simulink model "EarthmoverMechPT"  (Simulink 6.6)
settings: Solver=FixedStepDiscrete  StartTime=0  StopTime=100  FixedStep=0.01  MaxStep=0.01  RelTol=1e-12
undefined symbols (not defined in the file or in its folder): engineM, slippageM
libraries: simulink x17
settings Model: Creator=Messer  LastModifiedBy=Messer
settings SolverCC: SolverResetMethod=Robust
settings DebuggingCC: AlgebraicLoopMsg=none  SignalResolutionControl=TryResolveAllWithWarning  MultiTaskDSMMsg=warning  MultiTaskCondExecSysMsg=none  StrictBusMsg=None
settings RTWCC: IncludeERTFirstTime=on

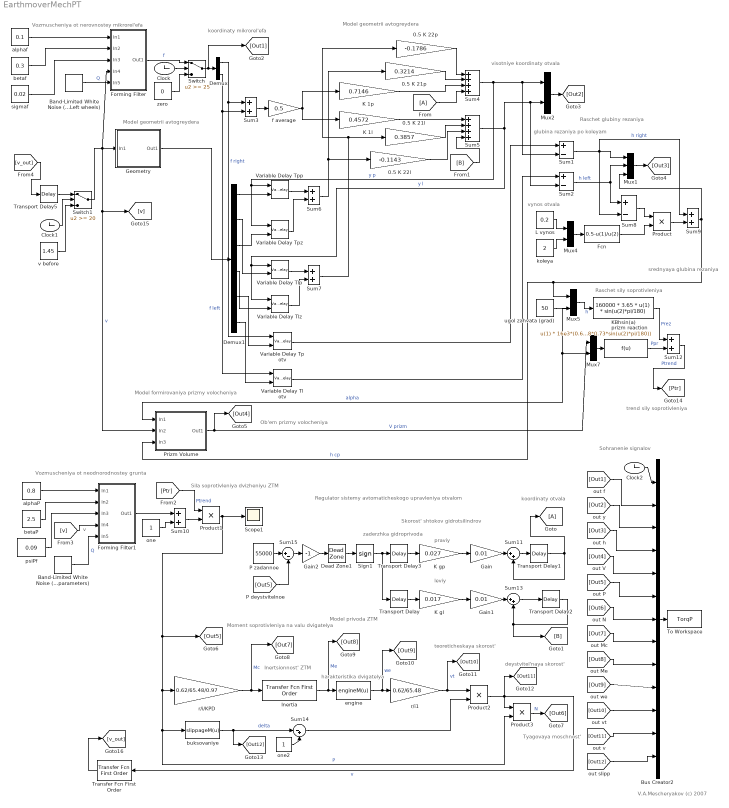
== system EarthmoverMechPT ==
  note: v
  note: V.A.Mescheryakov (c) 2007
  note: Sohranenie signalov
  note: Regulator sistemy
      | avtomaticheskogo upravleniya otvalom
  note: Skorost' shtokov
      | gidrotsilindrov
  note: praviy
  note: leviy
  note: zaderzhka
      | gidroprivoda
  note: Sila soprotivleniya
      | dvizheniyu ZTM
  note: harakteristika
      | dvigatelya
  note: Inertsionnost' ZTM
  note: Moment soprotivleniya
      | na valu dvigatelya
  note: Vozmuscheniya ot neodnorodnostey grunta
  note: teoreticheskaya skorost'
  note: deystvitel'naya skorost'
  note: koordinaty otvala
  note: Vozmuscheniya ot nerovnostey mikrorel'efa
  note: visotniye koordinaty otvala
  note: glubina rezaniya
      | po koleyam
  note: srednyaya
      | glubina
      | rezaniya
  note: vynos otvala
  note: trend sily soprotivleniya
  note: Ob'em prizmy volocheniya
  note: Model formirovaniya prizmy volocheniya
  note: Model geometrii avtogreydera
  note: Model geometrii avtogreydera
  note: koordinaty mikrorel'efa
  note: Model privoda ZTM
  note: Tyagovaya
      | moschnost'
  note: Raschet glubiny rezaniya
  note: Raschet sily soprotivleniya
  0.5 K 21l : Gain  Gain=0.3857
  0.5 K 21p : Gain  Gain=0.3214
  0.5 K 22l : Gain  Gain=-0.1143
  0.5 K 22p : Gain  Gain=-0.1786
  Band-Limited White Noise (Right & Left wheels) : simulink/Sources/Band-Limited White Noise  SystemSampleTime=-1  Cov=[1 1]  Ts=0.01  seed=[1111 2111]  VectorParams1D=off
  Band-Limited White Noise (Soil parameters) : simulink/Sources/Band-Limited White Noise  SystemSampleTime=-1  Cov=[1]  Ts=0.01  seed=[1112]
  Bus Creator2 : BusCreator  Inputs=13
  Clock : Clock
      settings: Decimation=10
  Clock1 : Clock
      settings: Decimation=10
  Clock2 : Clock
      settings: Decimation=10
  Dead Zone1 : DeadZone  LowerValue=-700  UpperValue=700  SaturateOnIntegerOverflow=on
  Demux : Demux  Outputs=2
  Demux1 : Demux  Outputs=6
  Fcn : Fcn  Expr=0.5-u(1)/u(2)
  Forming Filter : Subsystem
  Forming Filter1 : Subsystem
  Gain : Gain  Gain=0.01
  Gain1 : Gain  Gain=0.01
  Gain2 : Gain  Gain=-1
  Geometry : Subsystem
  Inertia : simulink/Discrete/Transfer Fcn First Order  SystemSampleTime=-1  PoleZ=exp(-1/0.48*0.01)  ICPrevOutput=0  DoSatur=off
  K 1l : Gain  Gain=0.4572
  K 1p : Gain  Gain=0.7146
  K gl : Gain  Gain=0.017
  K gp : Gain  Gain=0.027
  KBhsin(a) : Fcn  Expr=160000 * 3.65 * u(1) * sin(u(2)*pi/180)
  L vynos : Constant  Value=0.2
  Mux1 : Mux  Inputs=3
  Mux{2,4..5,7} (4 alike) : Mux  Inputs=2
  P zadannoe : Constant  Value=55000
  Prizm Volume : Subsystem
  Product{,1..3} (4 alike) : Product  RndMeth=Zero
  Scope1 : Scope
      settings: YMin=0  YMax=75000  SaveName=cr1  DataFormat=Array
  Sign1 : Signum
  Sum1 : Sum  Inputs=+-
  Sum{3,6..7,9..10,12} (6 alike) : Sum
  Sum11 : Sum  Inputs=|++
  Sum13 : Sum  Inputs=|++
  Sum14 : Sum  Inputs=|-+
  Sum15 : Sum  Inputs=|+-
  Sum2 : Sum  Inputs=+-
  Sum4 : Sum  Inputs=++++
  Sum5 : Sum  Inputs=++++
  Sum8 : Sum  Inputs=+-
  Switch : Switch  Threshold=25  ZeroCross=off
  Switch1 : Switch  Threshold=20  ZeroCross=off
  To Workspace : ToWorkspace  VariableName=TorqP  SampleTime=-1  SaveFormat=Array
  Transfer Fcn First Order : simulink/Discrete/Transfer Fcn First Order  Orientation=left  SystemSampleTime=-1  PoleZ=0.99  ICPrevOutput=0  DoSatur=off
  Transport Delay : TransportDelay  DelayTime=0.1  InitialOutput=-1
  Transport Delay1 : TransportDelay  DelayTime=0.01
  Transport Delay2 : TransportDelay  DelayTime=0.01
  Transport Delay3 : TransportDelay  DelayTime=0.1  InitialOutput=-1
  Transport Delay5 : TransportDelay  DelayTime=0.01  InitialOutput=1
  Variable Delay Tl otv : VariableTransportDelay  MaximumDelay=20
  Variable Delay Tlp : VariableTransportDelay  MaximumDelay=20
  Variable Delay Tlz : VariableTransportDelay  MaximumDelay=20
  Variable Delay Tp otv : VariableTransportDelay  MaximumDelay=20
  Variable Delay Tpp : VariableTransportDelay  MaximumDelay=20
  Variable Delay Tpz : VariableTransportDelay  MaximumDelay=20
  alphaP : Constant  Value=0.8
  alphaf : Constant  Value=0.1
  betaP : Constant  Value=2.5
  betaf : Constant  Value=0.3
  buksovaniye : MATLABFcn  MATLABFcn=slippageM(u)  OutputDimensions=1
  engine : MATLABFcn  MATLABFcn=engineM(u)  OutputDimensions=1
  f average : Gain  Gain=0.5
  koleya : Constant  Value=2
  one : Constant
  one2 : Constant
  prizm reaction : Fcn  Expr=u(1) * 16e3*(0.65*sin(u(2)*pi/180)+0.65*0.73*cos(u(2)*pi/180)+0.5868*0.73*sin(u(2)*pi/180))
  psiPf : Constant  Value=0.09
  r/i/KPD : Gain  Gain=0.62/65.48/0.97
  r/i1 : Gain  Gain=0.62/65.48
  sigmaf : Constant  Value=0.02
  ugol zahvata (grad) : Constant  Value=50
  v before : Constant  Value=1.45
  zero : Constant  Value=0
  wires:
  Forming Filter/1(Out1) -> Switch/1  "f"
  alphaf/1 -> Forming Filter/1(In1)
  betaf/1 -> Forming Filter/2(In2)
  sigmaf/1 -> Forming Filter/3(In3)
  Switch1/1 -> Forming Filter/4(In4), Geometry/1(In1), [v], Prizm Volume/2(In2)  "v"
  f average/1 -> K 1p/1, K 1l/1
  Geometry/1(Out1) -> Demux1/1
  Demux1/1 -> Variable Delay Tpp/2
  Demux1/2 -> Variable Delay Tlp/2
  Demux1/3 -> Variable Delay Tpz/2
  Demux1/4 -> Variable Delay Tlz/2
  Demux1/5 -> Variable Delay Tp otv/2
  Demux1/6 -> Variable Delay Tl otv/2
  Sum4/1 -> Variable Delay Tpz/1, Variable Delay Tpp/1, Sum1/2, Mux2/1  "y p"
  Sum5/1 -> Variable Delay Tlz/1, Variable Delay Tlp/1, Mux2/2, Sum2/2  "y l"
  K 1l/1 -> Sum5/1
  K 1p/1 -> Sum4/3
  Variable Delay Tpp/1 -> Sum6/1
  Variable Delay Tpz/1 -> Sum6/2
  Variable Delay Tlp/1 -> Sum7/1
  Variable Delay Tlz/1 -> Sum7/2
  0.5 K 21p/1 -> Sum4/2
  0.5 K 21l/1 -> Sum5/2
  Sum6/1 -> 0.5 K 21p/1, 0.5 K 22l/1
  Sum7/1 -> 0.5 K 21l/1, 0.5 K 22p/1
  0.5 K 22p/1 -> Sum4/1
  0.5 K 22l/1 -> Sum5/3
  Variable Delay Tp otv/1 -> Sum1/1
  Variable Delay Tl otv/1 -> Sum2/1
  Mux2/1 -> [Out2]
  [A] -> Sum4/4
  Sum1/1 -> Mux1/1, Sum8/2, Sum9/1  "h right"
  Sum2/1 -> Mux1/2, Sum8/1  "h left"
  Mux1/1 -> [Out3]
  Sum3/1 -> f average/1
  Clock/1 -> Switch/2
  zero/1 -> Switch/3
  [B] -> Sum5/4
  L vynos/1 -> Mux4/1
  koleya/1 -> Mux4/2
  Mux4/1 -> Fcn/1
  Sum8/1 -> Product/1
  Fcn/1 -> Product/2
  Product/1 -> Sum9/2
  Sum9/1 -> Mux1/3, Mux5/1, Prizm Volume/3(In3)  "h cp"
  ugol zahvata (grad)/1 -> Mux5/2, Mux7/2, Prizm Volume/1(In1)  "alpha"
  Mux5/1 -> KBhsin(a)/1  "h"
  KBhsin(a)/1 -> Sum12/1  "Prez"
  prizm reaction/1 -> Sum12/2  "Ppr"
  Mux7/1 -> prizm reaction/1
  Band-Limited White Noise (Right & Left wheels)/1 -> Forming Filter/5(In5)  "Q"
  Switch/1 -> Demux/1, [Out1]
  Demux/1 -> Sum3/1, Variable Delay Tp otv/1  "f right"
  Demux/2 -> Sum3/2, Variable Delay Tl otv/1  "f left"
  Prizm Volume/1(Out1) -> Mux7/1, [Out4]  "V prizm"
  alphaP/1 -> Forming Filter1/1(In1)
  betaP/1 -> Forming Filter1/2(In2)
  psiPf/1 -> Forming Filter1/3(In3)
  Band-Limited White Noise (Soil parameters)/1 -> Forming Filter1/5(In5)  "Q"
  one/1 -> Sum10/2
  Forming Filter1/1(Out1) -> Sum10/1
  Sum10/1 -> Product1/2
  Product1/1 -> r/i/KPD/1, Product3/2, buksovaniye/1, [Out5], Scope1/1  "P"
  K gp/1 -> Gain/1
  K gl/1 -> Gain1/1
  r/i1/1 -> Product2/1, [Out10]  "vt"
  Product2/1 -> [Out11], Product3/1, Transfer Fcn First Order/1  "v"
  Product3/1 -> [Out6]  "N"
  one2/1 -> Sum14/2
  Sum14/1 -> Product2/2
  r/i/KPD/1 -> Inertia/1, [Out7]  "Mc"
  Clock1/1 -> Switch1/2
  v before/1 -> Switch1/3
  Bus Creator2/1 -> To Workspace/1
  Clock2/1 -> Bus Creator2/1
  [Out1] -> Bus Creator2/2
  [Out2] -> Bus Creator2/3
  [Out3] -> Bus Creator2/4
  [Out4] -> Bus Creator2/5
  [Out5] -> Bus Creator2/6
  [Out6] -> Bus Creator2/7
  [Out7] -> Bus Creator2/8
  [Out8] -> Bus Creator2/9
  [Out9] -> Bus Creator2/10
  [Out10] -> Bus Creator2/11
  [Out11] -> Bus Creator2/12
  [Out12] -> Bus Creator2/13
  Inertia/1 -> engine/1, [Out8]  "Me"
  buksovaniye/1 -> Sum14/1, [Out12]  "delta"
  engine/1 -> r/i1/1, [Out9]  "we"
  Gain/1 -> Sum11/1
  Sum11/1 -> Transport Delay1/1
  Transport Delay1/1 -> Sum11/2, [A]
  Gain1/1 -> Sum13/1
  Sum13/1 -> Transport Delay2/1
  Transport Delay2/1 -> Sum13/2, [B]
  Sum12/1 -> [Ptr]  "Ptrend"
  [Ptr] -> Product1/1  "Ptrend"
  [v] -> Forming Filter1/4(In4)
  [v_out] -> Transport Delay5/1
  Transfer Fcn First Order/1 -> [v_out]
  Transport Delay5/1 -> Switch1/1
  P zadannoe/1 -> Sum15/1
  Dead Zone1/1 -> Sign1/1
  Sign1/1 -> Transport Delay3/1, Transport Delay/1
  Transport Delay3/1 -> K gp/1
  Transport Delay/1 -> K gl/1
  [Out5] -> Sum15/2
  Gain2/1 -> Dead Zone1/1
  Sum15/1 -> Gain2/1

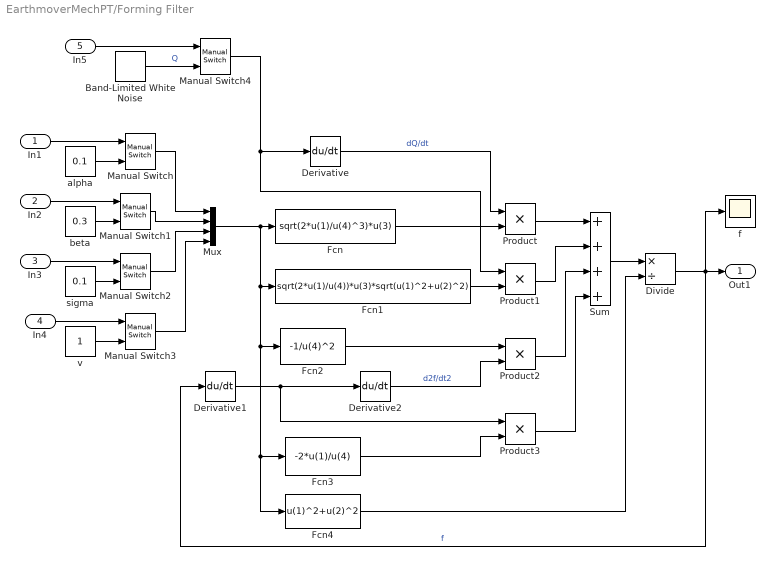
== system EarthmoverMechPT/Forming Filter ==
  In1 : Inport
  In2 : Inport  Port=2
  In3 : Inport  Port=3
  In4 : Inport  Port=4
  In5 : Inport  Port=5
  Band-Limited White Noise : simulink/Sources/Band-Limited White Noise  SystemSampleTime=-1  Cov=1  Ts=0.01  seed=[23341]
  Derivative : Derivative
  Derivative1 : Derivative
  Derivative2 : Derivative
  Divide : Product  Inputs=*/  OutScaling=2^-10
  Fcn : Fcn  Expr=sqrt(2*u(1)/u(4)^3)*u(3)
  Fcn1 : Fcn  Expr=sqrt(2*u(1)/u(4))*u(3)*sqrt(u(1)^2+u(2)^2)
  Fcn2 : Fcn  Expr=-1/u(4)^2
  Fcn3 : Fcn  Expr=-2*u(1)/u(4)
  Fcn4 : Fcn  Expr=u(1)^2+u(2)^2
  Manual Switch{,1..4} (5 alike) : simulink/Signal Routing/Manual Switch  SystemSampleTime=-1  sw=1  action=0  varsize=off
  Mux : Mux
  Product{,1..3} (4 alike) : Product  RndMeth=Zero
  Sum : Sum  Inputs=++++
  alpha : Constant  Value=0.1
  beta : Constant  Value=0.3
  f : Scope
      settings: SaveName=ScopeData12
  sigma : Constant  Value=0.1
  v : Constant
  Out1 : Outport
  wires:
  Mux/1 -> Fcn/1, Fcn1/1, Fcn3/1, Fcn4/1, Fcn2/1
  Derivative/1 -> Product/1  "dQ/dt"
  Fcn/1 -> Product/2
  Fcn1/1 -> Product1/2
  Product/1 -> Sum/1
  Product1/1 -> Sum/2
  Derivative1/1 -> Derivative2/1, Product3/1
  Derivative2/1 -> Product2/2  "d2f/dt2"
  Fcn2/1 -> Product2/1
  Product2/1 -> Sum/3
  Product3/1 -> Sum/4
  Fcn3/1 -> Product3/2
  Sum/1 -> Divide/1
  Fcn4/1 -> Divide/2
  Divide/1 -> Derivative1/1, f/1, Out1/1  "f"
  In1/1 -> Manual Switch/1
  alpha/1 -> Manual Switch/2
  Manual Switch/1 -> Mux/1
  In2/1 -> Manual Switch1/1
  beta/1 -> Manual Switch1/2
  Manual Switch1/1 -> Mux/2
  sigma/1 -> Manual Switch2/2
  In3/1 -> Manual Switch2/1
  Manual Switch2/1 -> Mux/3
  Manual Switch3/1 -> Mux/4
  In4/1 -> Manual Switch3/1
  v/1 -> Manual Switch3/2
  Band-Limited White Noise/1 -> Manual Switch4/2  "Q"
  In5/1 -> Manual Switch4/1
  Manual Switch4/1 -> Derivative/1, Product1/1

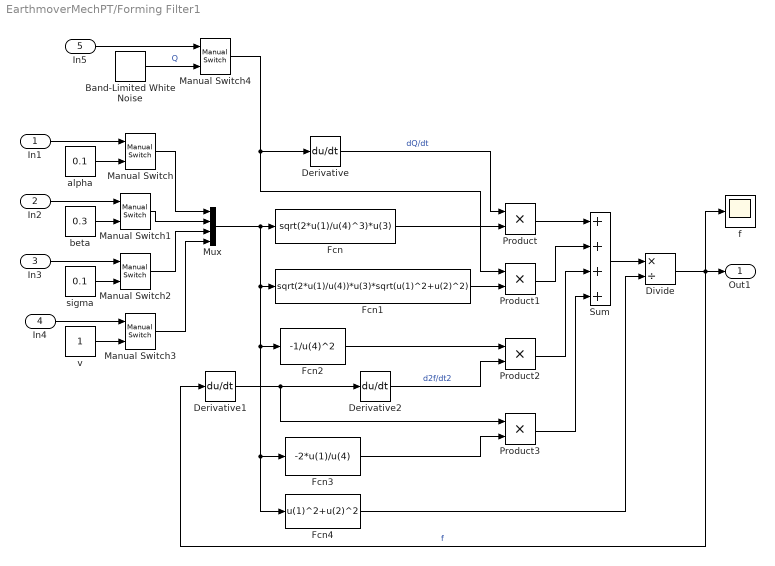
== system EarthmoverMechPT/Forming Filter1 ==
  In1 : Inport
  In2 : Inport  Port=2
  In3 : Inport  Port=3
  In4 : Inport  Port=4
  In5 : Inport  Port=5
  Band-Limited White Noise : simulink/Sources/Band-Limited White Noise  SystemSampleTime=-1  Cov=1  Ts=0.01  seed=[23341]
  Derivative : Derivative
  Derivative1 : Derivative
  Derivative2 : Derivative
  Divide : Product  Inputs=*/  OutScaling=2^-10
  Fcn : Fcn  Expr=sqrt(2*u(1)/u(4)^3)*u(3)
  Fcn1 : Fcn  Expr=sqrt(2*u(1)/u(4))*u(3)*sqrt(u(1)^2+u(2)^2)
  Fcn2 : Fcn  Expr=-1/u(4)^2
  Fcn3 : Fcn  Expr=-2*u(1)/u(4)
  Fcn4 : Fcn  Expr=u(1)^2+u(2)^2
  Manual Switch{,1..4} (5 alike) : simulink/Signal Routing/Manual Switch  SystemSampleTime=-1  sw=1  action=0  varsize=off
  Mux : Mux
  Product{,1..3} (4 alike) : Product  RndMeth=Zero
  Sum : Sum  Inputs=++++
  alpha : Constant  Value=0.1
  beta : Constant  Value=0.3
  f : Scope
      settings: SaveName=ScopeData12
  sigma : Constant  Value=0.1
  v : Constant
  Out1 : Outport
  wires:
  Mux/1 -> Fcn/1, Fcn1/1, Fcn3/1, Fcn4/1, Fcn2/1
  Derivative/1 -> Product/1  "dQ/dt"
  Fcn/1 -> Product/2
  Fcn1/1 -> Product1/2
  Product/1 -> Sum/1
  Product1/1 -> Sum/2
  Derivative1/1 -> Derivative2/1, Product3/1
  Derivative2/1 -> Product2/2  "d2f/dt2"
  Fcn2/1 -> Product2/1
  Product2/1 -> Sum/3
  Product3/1 -> Sum/4
  Fcn3/1 -> Product3/2
  Sum/1 -> Divide/1
  Fcn4/1 -> Divide/2
  Divide/1 -> Derivative1/1, f/1, Out1/1  "f"
  In1/1 -> Manual Switch/1
  alpha/1 -> Manual Switch/2
  Manual Switch/1 -> Mux/1
  In2/1 -> Manual Switch1/1
  beta/1 -> Manual Switch1/2
  Manual Switch1/1 -> Mux/2
  sigma/1 -> Manual Switch2/2
  In3/1 -> Manual Switch2/1
  Manual Switch2/1 -> Mux/3
  Manual Switch3/1 -> Mux/4
  In4/1 -> Manual Switch3/1
  v/1 -> Manual Switch3/2
  Band-Limited White Noise/1 -> Manual Switch4/2  "Q"
  In5/1 -> Manual Switch4/1
  Manual Switch4/1 -> Derivative/1, Product1/1

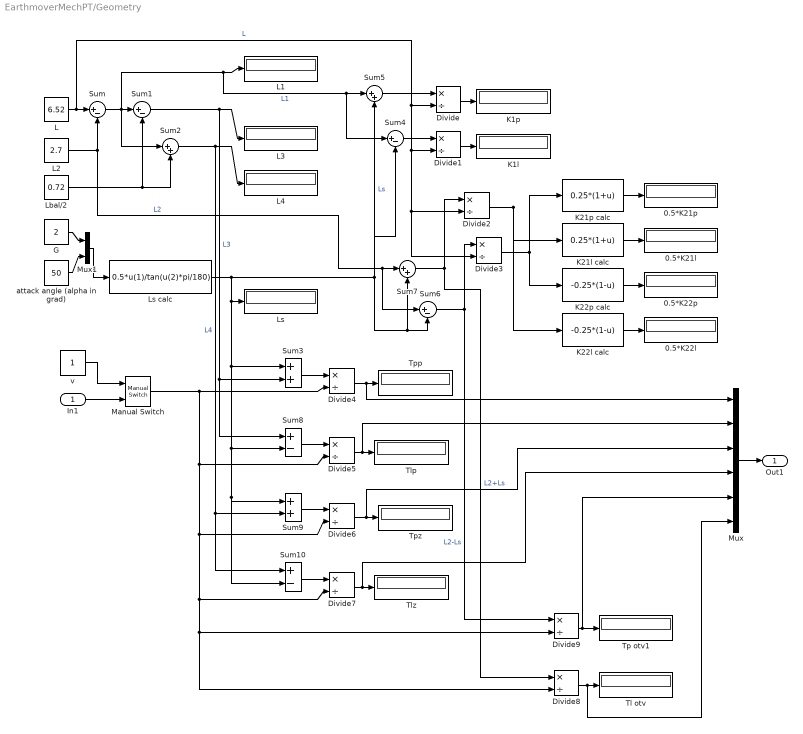
== system EarthmoverMechPT/Geometry ==
  In1 : Inport
  0.5*K21l : Display
  0.5*K21p : Display
  0.5*K22l : Display
  0.5*K22p : Display
  Divide{,1..9} (10 alike) : Product  Inputs=*/  OutScaling=2^-10
  G : Constant  Value=2
  K1l : Display
  K1p : Display
  K21l calc : Fcn  Expr=0.25*(1+u)
  K21p calc : Fcn  Expr=0.25*(1+u)
  K22l calc : Fcn  Expr=-0.25*(1-u)
  K22p calc : Fcn  Expr=-0.25*(1-u)
  L : Constant  Value=6.52
  L1 : Display
  L2 : Constant  Value=2.7
  L3 : Display
  L4 : Display
  Lbal/2 : Constant  Value=0.72
  Ls : Display
  Ls calc : Fcn  Expr=0.5*u(1)/tan(u(2)*pi/180)
  Manual Switch : simulink/Signal Routing/Manual Switch  SystemSampleTime=-1  sw=0  action=0  varsize=off
  Mux : Mux  Inputs=6
  Mux1 : Mux  Inputs=2
  Sum{,1,4,6} (4 alike) : Sum  Inputs=|+-
  Sum10 : Sum  Inputs=+-
  Sum2 : Sum  Inputs=|++
  Sum3 : Sum
  Sum5 : Sum  Inputs=|++
  Sum7 : Sum  Inputs=|++
  Sum8 : Sum  Inputs=+-
  Sum9 : Sum
  Tl otv : Display
  Tlp : Display
  Tlz : Display
  Tp otv1 : Display
  Tpp : Display
  Tpz : Display
  attack angle (alpha in grad) : Constant  Value=50
  v : Constant
  Out1 : Outport
  wires:
  L/1 -> Sum/1, Divide/2, Divide1/2, Divide2/2, Divide3/2  "L"
  L2/1 -> Sum/2, Sum7/1, Sum6/1  "L2"
  Sum/1 -> Sum2/1, Sum1/1, L1/1, Sum5/1, Sum4/1  "L1"
  Lbal/2/1 -> Sum1/2, Sum2/2
  Sum1/1 -> L3/1, Sum3/2, Sum8/1  "L3"
  Sum2/1 -> L4/1, Sum9/2, Sum10/1  "L4"
  G/1 -> Mux1/1
  Ls calc/1 -> Sum5/2, Sum4/2, Sum6/2, Sum7/2, Ls/1, Sum3/1, Sum8/2, Sum9/1, Sum10/2  "Ls"
  attack angle (alpha in grad)/1 -> Mux1/2
  Mux1/1 -> Ls calc/1
  Sum5/1 -> Divide/1
  Divide/1 -> K1p/1
  Sum4/1 -> Divide1/1
  Divide1/1 -> K1l/1
  Sum6/1 -> Divide3/1, Divide9/1  "L2-Ls"
  Sum7/1 -> Divide2/1, Divide8/1  "L2+Ls"
  K21p calc/1 -> 0.5*K21p/1
  K21l calc/1 -> 0.5*K21l/1
  K22p calc/1 -> 0.5*K22p/1
  K22l calc/1 -> 0.5*K22l/1
  Divide3/1 -> K21p calc/1, K22p calc/1
  Divide2/1 -> K22l calc/1, K21l calc/1
  Sum3/1 -> Divide4/1
  Manual Switch/1 -> Divide4/2, Divide5/2, Divide6/2, Divide7/2, Divide9/2, Divide8/2
  Sum8/1 -> Divide5/1
  Divide4/1 -> Tpp/1, Mux/1
  Divide5/1 -> Tlp/1, Mux/2
  Sum9/1 -> Divide6/1
  Sum10/1 -> Divide7/1
  Divide6/1 -> Tpz/1, Mux/3
  Divide7/1 -> Tlz/1, Mux/4
  Divide8/1 -> Tl otv/1, Mux/6
  Divide9/1 -> Tp otv1/1, Mux/5
  In1/1 -> Manual Switch/2
  v/1 -> Manual Switch/1
  Mux/1 -> Out1/1

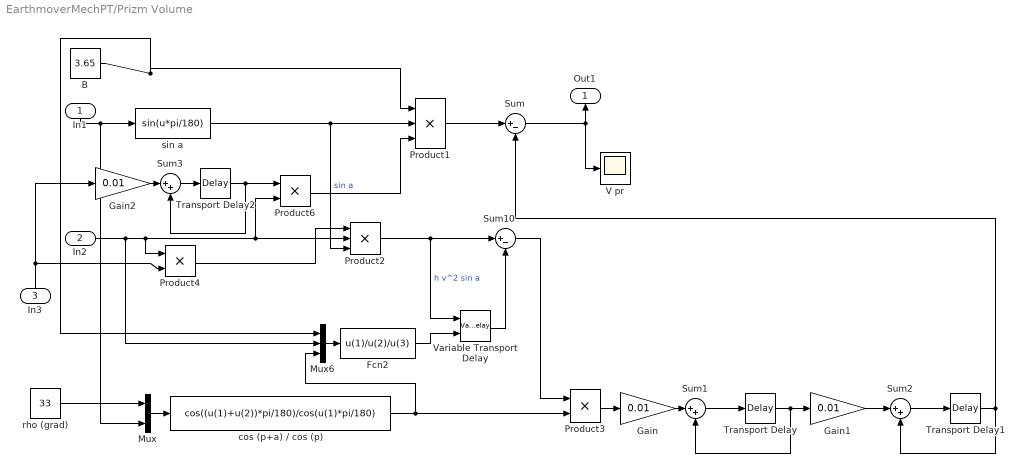
== system EarthmoverMechPT/Prizm Volume ==
  In1 : Inport  Orientation=down
  In2 : Inport  Port=2
  In3 : Inport  Orientation=up  Port=3
  B : Constant  Value=3.65
  Fcn2 : Fcn  Expr=u(1)/u(2)/u(3)
  Gain : Gain  Gain=0.01
  Gain1 : Gain  Gain=0.01
  Gain2 : Gain  Gain=0.01
  Mux : Mux  Inputs=2
  Mux6 : Mux  Inputs=3
  Product1 : Product  Inputs=3  RndMeth=Zero
  Product2 : Product  Inputs=3  RndMeth=Zero
  Product3 : Product  RndMeth=Zero
  Product4 : Product  RndMeth=Zero
  Product6 : Product  RndMeth=Zero
  Sum : Sum  Inputs=|+-
  Sum1 : Sum  Inputs=|++
  Sum10 : Sum  Inputs=|+-
  Sum2 : Sum  Inputs=|++
  Sum3 : Sum  Inputs=|++
  Transport Delay : TransportDelay  DelayTime=0.01
  Transport Delay1 : TransportDelay  DelayTime=0.01
  Transport Delay2 : TransportDelay  DelayTime=0.01
  V pr : Scope
      settings: YMin=0.4  YMax=2.7  SaveName=ScopeData4
  Variable Transport Delay : VariableTransportDelay  MaximumDelay=60
  cos (p+a) / cos (p) : Fcn  Expr=cos((u(1)+u(2))*pi/180)/cos(u(1)*pi/180)
  rho (grad) : Constant  Value=33
  sin a : Fcn  Expr=sin(u*pi/180)
  Out1 : Outport  Orientation=up
  wires:
  sin a/1 -> Product1/2, Product2/3  "sin a"
  B/1 -> Product1/1, Mux6/1
  Product1/1 -> Sum/1
  Mux/1 -> cos (p+a) / cos (p)/1
  rho (grad)/1 -> Mux/1
  Product2/1 -> Variable Transport Delay/1, Sum10/1  "h v^2 sin a"
  cos (p+a) / cos (p)/1 -> Product3/2, Mux6/3
  Variable Transport Delay/1 -> Sum10/2
  Fcn2/1 -> Variable Transport Delay/2
  Mux6/1 -> Fcn2/1
  Sum10/1 -> Product3/1
  Product4/1 -> Product2/1
  Product6/1 -> Product1/3
  Sum/1 -> V pr/1, Out1/1
  In1/1 -> Mux/2, sin a/1
  In2/1 -> Mux6/2, Product4/1, Product2/2, Product6/2
  In3/1 -> Product4/2, Gain2/1
  Gain/1 -> Sum1/1
  Sum1/1 -> Transport Delay/1
  Transport Delay/1 -> Sum1/2, Gain1/1
  Gain1/1 -> Sum2/1
  Sum2/1 -> Transport Delay1/1
  Transport Delay1/1 -> Sum2/2, Sum/2
  Product3/1 -> Gain/1
  Gain2/1 -> Sum3/1
  Sum3/1 -> Transport Delay2/1
  Transport Delay2/1 -> Sum3/2, Product6/1
